simulink model "heatex_sim_original"  (R2020a)
settings: Solver=ode4  StartTime=0.0  StopTime=200  FixedStep=2  RelTol=1e-3  EnableMultiTasking=on
libraries: cstblocks x4
settings Model: Creator=The MathWorks, Inc.  LastModifiedBy=nikhil
settings DataIOCC: LimitDataPoints=on  SaveFormat=Array  SaveOutput=off  SaveTime=off  ReturnWorkspaceOutputs=off
settings OptimizationCC: BlockReduction=off  BooleanDataType=off  InitFltsAndDblsToZero=on  LifeSpan=inf
settings DebuggingCC: SaveWithParameterizedLinksMsg=none  UnderspecifiedInitializationDetection=Classic  MergeDetectMultiDrivingBlocksExec=none  SignalResolutionControl=TryResolveAllWithWarning  MultiTaskDSMMsg=warning  MultiTaskCondExecSysMsg=none  FcnCallInpInsideContextMsg=warning  StateNameClashWarn=warning  SFUnexpectedBacktrackingDiag=warning  SFNoUnconditionalDefaultTransitionDiag=warning  SFExecutionAtInitializationDiag=none  ArithmeticOperatorsInVariantConditions=warning
settings HardwareCC: ProdBitPerPointer=32  ProdBitPerSizeT=32  ProdBitPerPtrDiffT=32  ProdLargestAtomicFloat=None  ProdIntDivRoundTo=Undefined  ProdEndianess=Unspecified  ProdWordSize=32  ProdHWDeviceType=32-bit Generic  TargetUnknown=on
settings ModelReferenceCC: PropagateSignalLabelsOutOfModel=off
settings SFSimCC: SimUseLocalCustomCode=off  CustomCodeUndefinedFunction=UseInterfaceOnly
settings RTWCC: RTWUseLocalCustomCode=off
settings CodeAppCC: StateflowObjectComments=on
settings GRTTargetCC: TargetFcnLib=ansi_tfl_tmw.mat  TargetLangStandard=C89/C90 (ANSI)  CombineOutputUpdateFcns=off  GRTInterface=on
settings ConfigComp: CovMetricSettings=dw  CovHtmlReporting=on  CovSaveCumulativeToWorkspaceVar=on  CovSaveSingleToWorkspaceVar=on  CovExternalEMLEnable=off

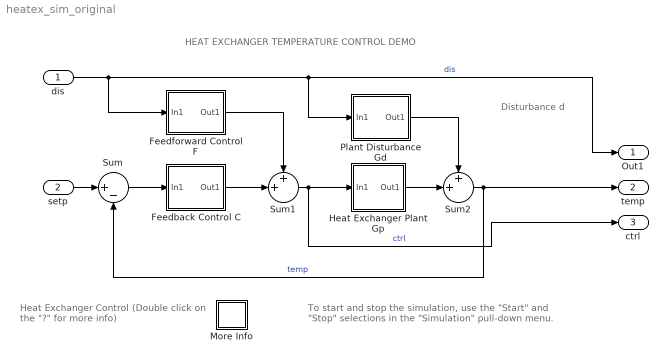
== system heatex_sim_original ==
  note: HEAT EXCHANGER TEMPERATURE CONTROL DEMO
  note: Disturbance d
  note: Heat Exchanger Control
      | (Double click on the "?" for more info)
  note: To start and stop the simulation, use the "Start" and
      | "Stop" selections in the "Simulation" pull-down menu.
  dis : Inport
  setp : Inport  Port=2
  Feedback Control C : Subsystem
  Feedforward Control F : Subsystem
  Heat Exchanger Plant Gp : Subsystem
  More Info : Subsystem
      mask Display: disp('?')
  Plant Disturbance Gd : Subsystem
  Sum : Sum  Inputs=|+-  InputSameDT=on  SaturateOnIntegerOverflow=on  OutDataTypeStr=Inherit: Same as first input
  Sum1 : Sum  Inputs=++|  InputSameDT=on  SaturateOnIntegerOverflow=on  OutDataTypeStr=Inherit: Same as first input
  Sum2 : Sum  Inputs=++|  InputSameDT=on  SaturateOnIntegerOverflow=on  OutDataTypeStr=Inherit: Same as first input
  Out1 : Outport
  temp : Outport  Port=2
  ctrl : Outport  Port=3
  wires:
  setp/1 -> Sum/1
  Sum/1 -> Feedback Control C/1(In1)
  Sum1/1 -> ctrl/1, Heat Exchanger Plant Gp/1(In1)  "ctrl"
  Sum2/1 -> temp/1, Sum/2  "temp"
  Feedforward Control F/1(Out1) -> Sum1/1
  dis/1 -> Feedforward Control F/1(In1), Out1/1, Plant Disturbance Gd/1(In1)  "dis"
  Feedback Control C/1(Out1) -> Sum1/2
  Heat Exchanger Plant Gp/1(Out1) -> Sum2/2
  Plant Disturbance Gd/1(Out1) -> Sum2/1

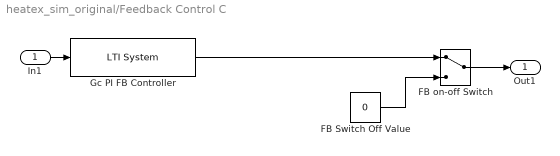
== system heatex_sim_original/Feedback Control C ==
  In1 : Inport
  FB Switch Off Value : Constant  Value=0
  FB on-off Switch : ManualSwitch
      settings: OpenFcn=manswitch('Open');heatex_clbk('FBSelect')
  Gc PI FB Controller : cstblocks/LTI System  sys=tf([30.31 1.23],[24.56 0])  IC=[]
  Out1 : Outport
  wires:
  In1/1 -> Gc PI FB Controller/1
  Gc PI FB Controller/1 -> FB on-off Switch/1
  FB on-off Switch/1 -> Out1/1
  FB Switch Off Value/1 -> FB on-off Switch/2

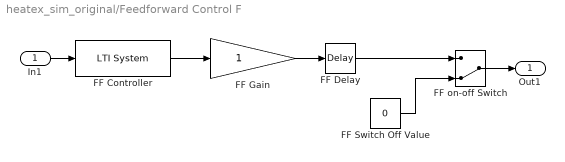
== system heatex_sim_original/Feedforward Control F ==
  In1 : Inport
  FF Controller : cstblocks/LTI System  sys=tf(-[21.3 1],[25 1])  IC=[]
  FF Delay : TransportDelay  DelayTime=25
      settings: CloseFcn=disp('hello')
  FF Gain : Gain  SaturateOnIntegerOverflow=on  OutDataTypeStr=Inherit: Same as input  ParamDataTypeStr=Inherit: Same as input
      settings: CloseFcn=disp('hello')
  FF Switch Off Value : Constant  Value=0
  FF on-off Switch : ManualSwitch  CurrentSetting=0
      settings: OpenFcn=manswitch('Open');heatex_clbk('FFSelect')
  Out1 : Outport
  wires:
  In1/1 -> FF Controller/1
  FF Gain/1 -> FF Delay/1
  FF Controller/1 -> FF Gain/1
  FF Delay/1 -> FF on-off Switch/1
  FF on-off Switch/1 -> Out1/1
  FF Switch Off Value/1 -> FF on-off Switch/2

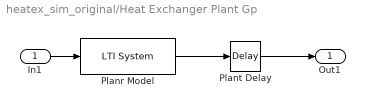
== system heatex_sim_original/Heat Exchanger Plant Gp ==
  In1 : Inport
  Planr Model : cstblocks/LTI System  sys=tf(1,[21.3 1])  IC=[]
  Plant Delay : TransportDelay  DelayTime=14.7
  Out1 : Outport
  wires:
  In1/1 -> Planr Model/1
  Planr Model/1 -> Plant Delay/1
  Plant Delay/1 -> Out1/1

== system heatex_sim_original/More Info ==
  note: Try experimenting with switching between
      | using Feedforward and/or Feedback control.
      | Type heatex at the MATLAB prompt to see the demo.
  note: This demonstration shows the temperature control of a continuous stirred
      | tank reactor (CSTR) using a heat exchanger.
      | The controllers have been designed to regulate the temperature of the
      | liquid in the tank when subject to disturbances in the temperature of inlet flow.

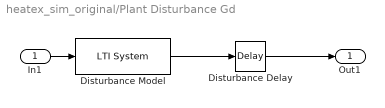
== system heatex_sim_original/Plant Disturbance Gd ==
  In1 : Inport
  Disturbance Delay : TransportDelay  DelayTime=35
  Disturbance Model : cstblocks/LTI System  sys=tf(1,[25 1])  IC=[]
  Out1 : Outport
  wires:
  Disturbance Delay/1 -> Out1/1
  In1/1 -> Disturbance Model/1
  Disturbance Model/1 -> Disturbance Delay/1
